simulink model "PIDimc"  (R2020a)
settings: Solver=VariableStepAuto  StartTime=0.0  StopTime=15  RelTol=1e-5
settings Model: Creator=batis  LastModifiedBy=batis

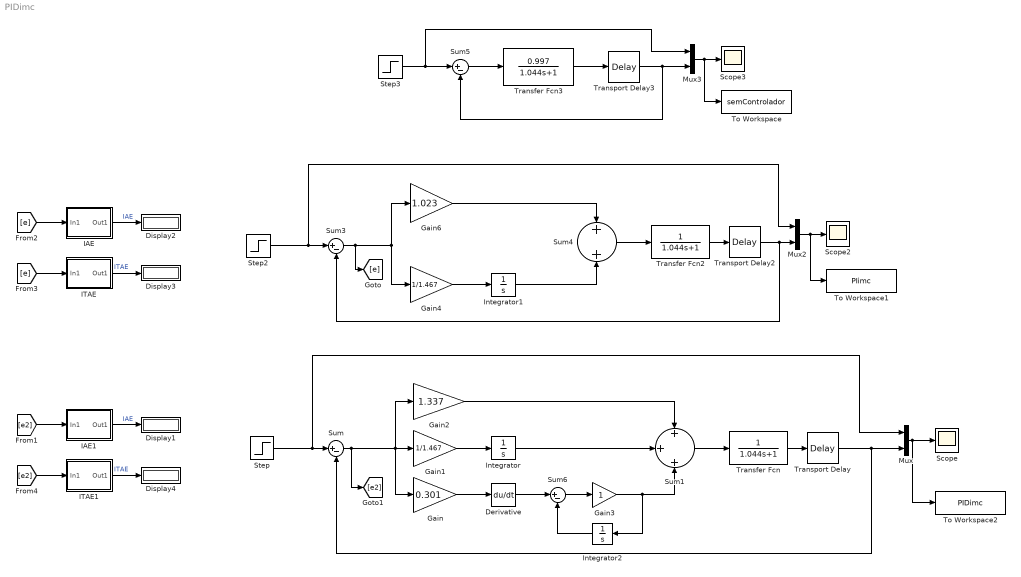
== system PIDimc ==
  Derivative : Derivative
  Display{1..4} (4 alike) : Display
  Gain : Gain  Gain=0.301
  Gain1 : Gain  Gain=1/1.467
  Gain2 : Gain  Gain=1.337
  Gain3 : Gain
  Gain4 : Gain  Gain=1/1.467
  Gain6 : Gain  Gain=1.023
  IAE : Subsystem
  IAE1 : Subsystem
  ITAE : Subsystem
  ITAE1 : Subsystem
  Integrator : Integrator
  Integrator1 : Integrator
  Integrator2 : Integrator
  Mux : Mux  Inputs=2
  Mux2 : Mux  Inputs=2
  Mux3 : Mux  Inputs=2
  Scope : Scope
  Scope2 : Scope
  Scope3 : Scope
  Step : Step  After=3  SampleTime=0
  Step2 : Step  After=3  SampleTime=0
  Step3 : Step  After=3  SampleTime=0
  Sum{,3,5..6} (4 alike) : Sum  Inputs=|+-
  Sum1 : Sum  Inputs=+|+|+
  Sum4 : Sum  Inputs=+|+
  To Workspace : ToWorkspace  VariableName=semControlador  SaveFormat=Structure With Time  SampleTime=-1
  To Workspace1 : ToWorkspace  VariableName=PIimc  SaveFormat=Structure With Time  SampleTime=-1
  To Workspace2 : ToWorkspace  VariableName=PIDimc  SaveFormat=Structure With Time  SampleTime=-1
  Transfer Fcn : TransferFcn  Denominator=[1.044 1]
  Transfer Fcn2 : TransferFcn  Denominator=[1.044 1]
  Transfer Fcn3 : TransferFcn  Numerator=[0.997]  Denominator=[1.044 1]
  Transport Delay : TransportDelay  DelayTime=0.846
  Transport Delay2 : TransportDelay  DelayTime=0.846
  Transport Delay3 : TransportDelay  DelayTime=0.846  FixedBuffer=on
  wires:
  Sum/1 -> [e2], Gain/1, Gain2/1, Gain1/1
  Sum1/1 -> Transfer Fcn/1
  Step/1 -> Sum/1, Mux/1
  Mux/1 -> To Workspace2/1, Scope/1
  Gain/1 -> Derivative/1
  Transfer Fcn/1 -> Transport Delay/1
  Transport Delay/1 -> Mux/2, Sum/2
  Gain2/1 -> Sum1/1
  Gain1/1 -> Integrator/1
  Integrator/1 -> Sum1/2
  Gain6/1 -> Sum4/1
  Transport Delay2/1 -> Mux2/2, Sum3/2
  Mux2/1 -> To Workspace1/1, Scope2/1
  Sum3/1 -> [e], Gain6/1, Gain4/1
  Gain4/1 -> Integrator1/1
  Transfer Fcn2/1 -> Transport Delay2/1
  Integrator1/1 -> Sum4/2
  Sum4/1 -> Transfer Fcn2/1
  Step2/1 -> Mux2/1, Sum3/1
  Transport Delay3/1 -> Mux3/2, Sum5/2
  Step3/1 -> Sum5/1, Mux3/1
  Transfer Fcn3/1 -> Transport Delay3/1
  Mux3/1 -> To Workspace/1, Scope3/1
  Sum5/1 -> Transfer Fcn3/1
  Derivative/1 -> Sum6/1
  Sum6/1 -> Gain3/1
  Gain3/1 -> Integrator2/1, Sum1/3
  Integrator2/1 -> Sum6/2
  [e] -> ITAE/1(In1)
  IAE/1(Out1) -> Display2/1  "IAE"
  [e] -> IAE/1(In1)
  ITAE/1(Out1) -> Display3/1  "ITAE"
  ITAE1/1(Out1) -> Display4/1  "ITAE"
  [e2] -> IAE1/1(In1)
  IAE1/1(Out1) -> Display1/1  "IAE"
  [e2] -> ITAE1/1(In1)

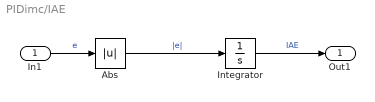
== system PIDimc/IAE ==
  In1 : Inport
  Abs : Abs
  Integrator : Integrator
  Out1 : Outport
  wires:
  Integrator/1 -> Out1/1  "IAE"
  In1/1 -> Abs/1  "e"
  Abs/1 -> Integrator/1  "|e|"

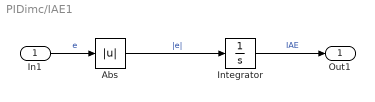
== system PIDimc/IAE1 ==
  In1 : Inport
  Abs : Abs
  Integrator : Integrator
  Out1 : Outport
  wires:
  Integrator/1 -> Out1/1  "IAE"
  In1/1 -> Abs/1  "e"
  Abs/1 -> Integrator/1  "|e|"

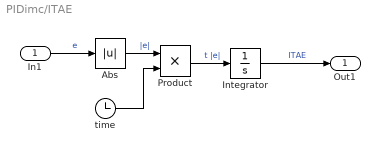
== system PIDimc/ITAE ==
  In1 : Inport
  Abs : Abs
  Integrator : Integrator
  Product : Product
  time : Clock
  Out1 : Outport
  wires:
  In1/1 -> Abs/1  "e"
  Integrator/1 -> Out1/1  "ITAE"
  time/1 -> Product/2
  Abs/1 -> Product/1  "|e|"
  Product/1 -> Integrator/1  "t |e|"

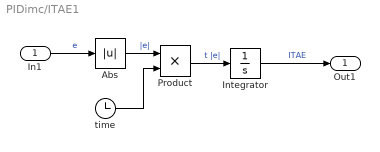
== system PIDimc/ITAE1 ==
  In1 : Inport
  Abs : Abs
  Integrator : Integrator
  Product : Product
  time : Clock
  Out1 : Outport
  wires:
  In1/1 -> Abs/1  "e"
  Integrator/1 -> Out1/1  "ITAE"
  time/1 -> Product/2
  Abs/1 -> Product/1  "|e|"
  Product/1 -> Integrator/1  "t |e|"
